simulink model "MergedPic"  (R2025a)
settings: Solver=FixedStepDiscrete  StartTime=0.0  StopTime=inf  FixedStep=0.001  RelTol=1e-3
settings Model: Creator=kevin  LastModifiedBy=kevin

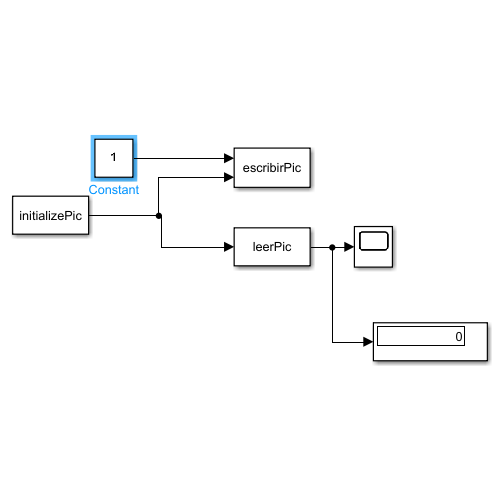
[thumbnail: Simulink's stored preview of the top-level diagram]
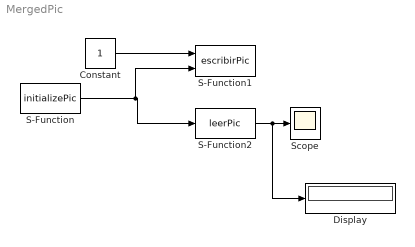
== system MergedPic ==
  Constant : Constant
  Display : Display
  S-Function : S-Function  FunctionName=initializePic  SFunctionDeploymentMode=off  EnableBusSupport=off
  S-Function1 : S-Function  FunctionName=escribirPic  SFunctionDeploymentMode=off  EnableBusSupport=off
  S-Function2 : S-Function  FunctionName=leerPic  SFunctionDeploymentMode=off  EnableBusSupport=off
  Scope : Scope
      settings: ActiveDisplayYMinimum=-1  ActiveDisplayYMaximum=1
  wires:
  S-Function/1 -> S-Function1/2, S-Function2/1
  Constant/1 -> S-Function1/1
  S-Function2/1 -> Display/1, Scope/1
